simulink model "Vaja6_simulink"  (R2019b)
settings: Solver=FixedStepDiscrete  StartTime=0.0  StopTime=8  FixedStep=dT  RelTol=1e-3  EnableMultiTasking=on
values from neighbouring files (symbols this model uses):
  dT = 1/500    (= 0.002)    [initVR.m]    (also in trajectory.m = 0.00025)
  q0 = [0 0 0 0 90 0]'*pi/180    [initVR.m]    (also in trajectory.m)
undefined symbols (not defined in the file or in its folder): DiscIntNeverNeededParam, q2ZYXeul
libraries: simulink x2, xpcutilitieslib x2, dspnetwork x2, dspinverses x1
Description:
  | Real-Time Van der Pol Simulation
  | 
  | This demonstration shows a real-time version of the Simulink Van der Pol
  | simulation demo. This model does not need any external signals, so it does
  | not need any data acquisition hardware or driver. This makes the model ideal
  | for first experiments with Real-Time Windows Target, without need to
  | worry about proper I/O hardware configuration.
  | 
  | How to run this demo:
  | 
  |   1. Build the model using Tools -> Real-Time Workshop -> Build Model.
  |   2. Connect to the real-time code using Simulation -> Connect to target.
  |   3. Start the real-time execution using Simulation -> Start real-time code.
settings Model: EnablePacing=on  Creator=Houska  LastModifiedBy=student
settings DataIOCC: LimitDataPoints=on  SaveFormat=Array  SignalLoggingSaveFormat=ModelDataLogs  SaveOutput=off  SaveTime=off  ReturnWorkspaceOutputs=off  SignalLoggingName=logsOut
settings OptimizationCC: ExpressionDepthLimit=2147483647  InitFltsAndDblsToZero=on  LifeSpan=inf
settings DebuggingCC: SaveWithParameterizedLinksMsg=none  UnderspecifiedInitializationDetection=Classic  MergeDetectMultiDrivingBlocksExec=none  SignalResolutionControl=TryResolveAllWithWarning  MultiTaskDSMMsg=warning  MultiTaskCondExecSysMsg=none  FcnCallInpInsideContextMsg=warning  StateNameClashWarn=warning  SFUnexpectedBacktrackingDiag=warning  SFNoUnconditionalDefaultTransitionDiag=warning  SFExecutionAtInitializationDiag=none  ArithmeticOperatorsInVariantConditions=warning
settings HardwareCC: ProdBitPerPointer=32  ProdBitPerSizeT=32  ProdBitPerPtrDiffT=32  ProdLargestAtomicFloat=None  ProdWordSize=32  ProdHWDeviceType=32-bit Real-Time Windows Target
settings ModelReferenceCC: PropagateSignalLabelsOutOfModel=off
settings SFSimCC: SimUseLocalCustomCode=off  SimParseCustomCode=off  CustomCodeUndefinedFunction=UseInterfaceOnly
settings RTWCC: Description=Real-Time Windows Target  SystemTargetFile=rtwin.tlc  TemplateMakefile=rtwin.tmf  RTWUseLocalCustomCode=off
settings CodeAppCC: StateflowObjectComments=on
settings TargetCC: TargetFcnLib=ansi_tfl_tmw.mat  ModelReferenceCompliant=off  CompOptLevelCompliant=off  PreserveStateflowLocalDataDimensions=off
settings ConfigComp: CovMetricSettings=dw  CovHtmlReporting=on  CovSaveCumulativeToWorkspaceVar=on  CovSaveSingleToWorkspaceVar=on  CovExternalEMLEnable=off

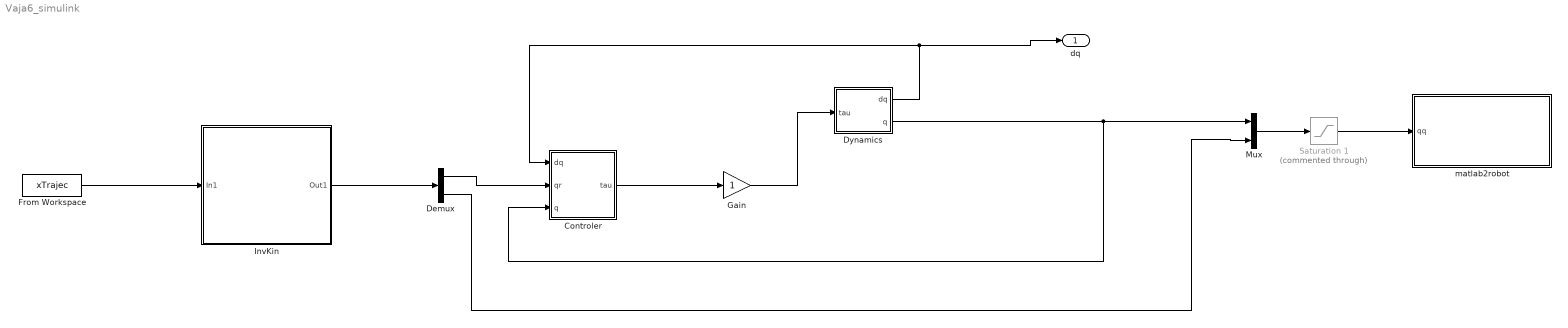
== system Vaja6_simulink ==
  Controler : Subsystem
  Demux : Demux  Outputs=2
  Dynamics : Subsystem
  From Workspace : FromWorkspace  VariableName=xTrajec  SampleTime=0
  Gain : Gain
  InvKin : Subsystem
  Mux : Mux  Inputs=2
  Saturation 1 : Saturate  Commented=through
  matlab2robot : Subsystem  mask{selUDP=Simulacija, slrt_ip='192.168.65.250', slrt_port=55555, sampleTime=dT}
      mask prompts: selUDP "Izvajanje programa:"; slrt_ip "Simulink Real Time IP:"; slrt_port "Simulink Real Time Port:"; sampleTime "Vzorcni cas:"
      mask init:
      | switch selUDP
      |     case 1
      |         enSim = 1;
      |         enRob = 0;
      |     case 2
      |         enSim = 0;
      |         enRob = 1;
      |     otherwise
      |         enSim = 0;
      |         enRob = 0;
      | end
      mask TypeOptions selUDP: Simulacija | Robot
  dq : Outport
  wires:
  Saturation 1/1 -> matlab2robot/1(qq)
  From Workspace/1 -> InvKin/1(In1)
  Dynamics/2(q) -> Mux/1, Controler/3(q)
  Controler/1(tau) -> Gain/1
  Dynamics/1(dq) -> Controler/1(dq), dq/1
  InvKin/1(Out1) -> Demux/1
  Demux/1 -> Controler/2(qr)
  Mux/1 -> Saturation 1/1
  Demux/2 -> Mux/2
  Gain/1 -> Dynamics/1(tau)

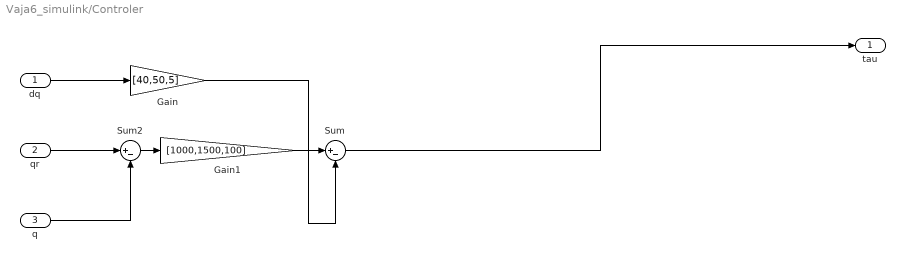
== system Vaja6_simulink/Controler ==
  dq : Inport
  qr : Inport  Port=2
  q : Inport  Port=3
  Gain : Gain  Gain=[40,50,5]
  Gain1 : Gain  Gain=[1000,1500,100]
  Sum : Sum  Inputs=|+-
  Sum2 : Sum  Inputs=|+-
  tau : Outport
  wires:
  Sum/1 -> tau/1
  Sum2/1 -> Gain1/1
  q/1 -> Sum2/2
  dq/1 -> Gain/1
  qr/1 -> Sum2/1
  Gain/1 -> Sum/2
  Gain1/1 -> Sum/1

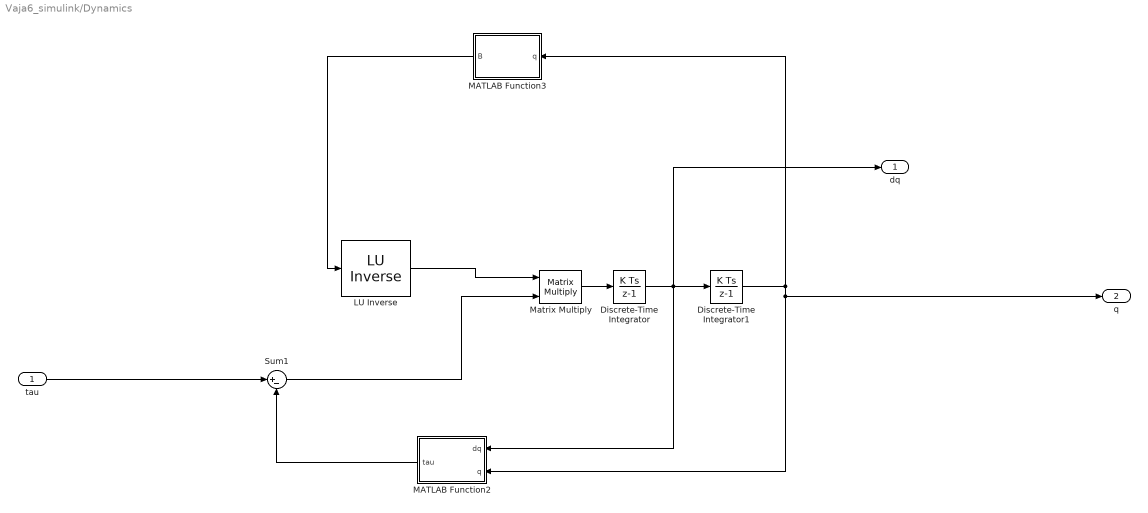
== system Vaja6_simulink/Dynamics ==
  tau : Inport
  " LU Inverse" : dspinverses/ LU Inverse
      settings: SourceProductName=DSP System Toolbox
  Discrete-Time Integrator : DiscreteIntegrator  InitialCondition=[0 0 0]  SampleTime=dT  ICPrevOutput=DiscIntNeverNeededParam  ICPrevScaledInput=DiscIntNeverNeededParam
  Discrete-Time Integrator1 : DiscreteIntegrator  InitialCondition=q0(1:3)  SampleTime=dT  ICPrevOutput=DiscIntNeverNeededParam  ICPrevScaledInput=DiscIntNeverNeededParam
  MATLAB Function2 : MATLAB Function  TreatAsAtomicUnit=on
  MATLAB Function3 : MATLAB Function  TreatAsAtomicUnit=on
  Matrix Multiply : Product  Multiplication=Matrix(*)
  Sum1 : Sum  Inputs=|+-
  dq : Outport
  q : Outport  Port=2
  wires:
  Discrete-Time Integrator/1 -> dq/1, Discrete-Time Integrator1/1, MATLAB Function2/1(dq)
  Discrete-Time Integrator1/1 -> q/1, MATLAB Function2/2(q), MATLAB Function3/1(q)
  Sum1/1 -> Matrix Multiply/2
  MATLAB Function3/1(B) -> " LU Inverse"/1
  " LU Inverse"/1 -> Matrix Multiply/1
  MATLAB Function2/1(tau) -> Sum1/2
  Matrix Multiply/1 -> Discrete-Time Integrator/1
  tau/1 -> Sum1/1

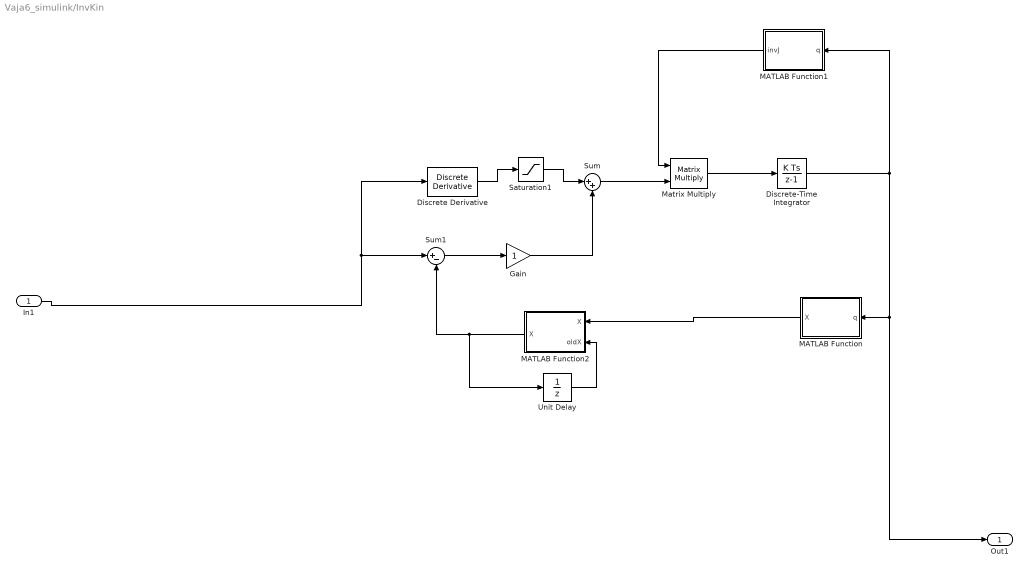
== system Vaja6_simulink/InvKin ==
  In1 : Inport
  Discrete Derivative : simulink/Discrete/Discrete Derivative  gainval=1.0  ICPrevScaledInput=0.0  OutMin=[]  OutMax=[]  OutDataType=fixdt(1, 16)  OutScaling=2^-10  DoSatur=off
  Discrete-Time Integrator : DiscreteIntegrator  InitialCondition=q0  SampleTime=dT  ICPrevOutput=DiscIntNeverNeededParam  ICPrevScaledInput=DiscIntNeverNeededParam
  Gain : Gain
  MATLAB Function : MATLAB Function  TreatAsAtomicUnit=on
  MATLAB Function1 : MATLAB Function  TreatAsAtomicUnit=on
  MATLAB Function2 : MATLAB Function  TreatAsAtomicUnit=on
  Matrix Multiply : Product  Multiplication=Matrix(*)
  Saturation1 : Saturate
  Sum : Sum  Inputs=|++
  Sum1 : Sum  Inputs=|+-
  Unit Delay : UnitDelay  InitialCondition=q2ZYXeul(q0)  SampleTime=-1  HasFrameUpgradeWarning=on
  Out1 : Outport
  wires:
  Sum1/1 -> Gain/1
  Saturation1/1 -> Sum/1
  MATLAB Function/1(X) -> MATLAB Function2/1("X ")
  Unit Delay/1 -> MATLAB Function2/2(oldX)
  MATLAB Function2/1(X) -> Unit Delay/1, Sum1/2
  Sum/1 -> Matrix Multiply/2
  Gain/1 -> Sum/2
  Matrix Multiply/1 -> Discrete-Time Integrator/1
  In1/1 -> Discrete Derivative/1, Sum1/1
  MATLAB Function1/1(invJ) -> Matrix Multiply/1
  Discrete-Time Integrator/1 -> Out1/1, MATLAB Function/1(q), MATLAB Function1/1(q)
  Discrete Derivative/1 -> Saturation1/1

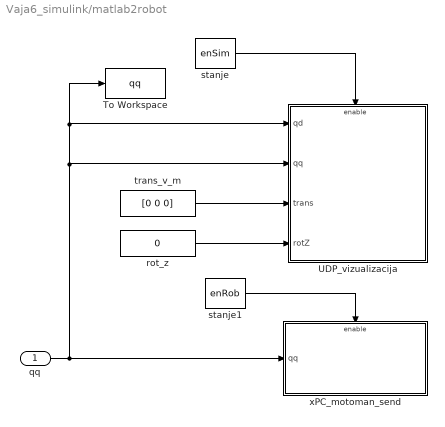
== system Vaja6_simulink/matlab2robot ==
  qq : Inport
  To Workspace : ToWorkspace  VariableName=qq  SampleTime=-1
  UDP_vizualizacija : Subsystem
  rot_z : Constant  Value=0
  stanje : Constant  Value=enSim  SampleTime=dT
  stanje1 : Constant  Value=enRob  SampleTime=dT
  trans_v_m : Constant  Value=[0 0 0]
  xPC_motoman_send : Subsystem  mask{IDSeje=rand(1), GetReady=1, slrt_ip1=slrt_ip, slrt_port1=slrt_port}
      mask prompts: IDSeje "IDSeje Function"; GetReady "GetReady Function"; slrt_ip1 "xPC Target IP"; slrt_port1 "xPC Target port"
      mask init:
      | %set_param([gcb,'/Send'],'remoteURL',slrt_ip1);
      | %set_param([gcb,'/Send'],'remotePort',num2str(slrt_port1));
      mask Callback slrt_port1: % set_param([gcb,'/Send'],'ipPort',slrt_port)
  wires:
  stanje/1 -> UDP_vizualizacija/Enable
  rot_z/1 -> UDP_vizualizacija/4(rotZ)
  trans_v_m/1 -> UDP_vizualizacija/3(trans)
  qq/1 -> To Workspace/1, UDP_vizualizacija/1(qd), UDP_vizualizacija/2(qq), xPC_motoman_send/1(qq)
  stanje1/1 -> xPC_motoman_send/Enable

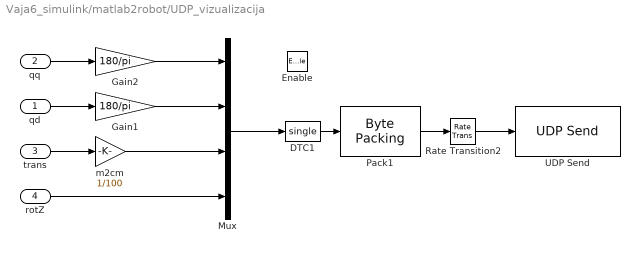
== system Vaja6_simulink/matlab2robot/UDP_vizualizacija ==
  qd : Inport
  qq : Inport  Port=2
  trans : Inport  Port=3
  rotZ : Inport  Port=4
  Enable : EnablePort  StatesWhenEnabling=reset
  DTC1 : DataTypeConversion  OutDataTypeStr=single
  Gain1 : Gain  Gain=180/pi
  Gain2 : Gain  Gain=180/pi
  Mux : Mux
  Pack1 : xpcutilitieslib/Byte Packing   MaskPackedDataType=uint8  MaskUnpackedDataTypes={'single'}  MaskAlignment=1
  Rate Transition2 : RateTransition
  UDP Send : dspnetwork/UDP Send  remoteURL='127.0.0.1'  remotePort=25300  localURL='0.0.0.0'  localPortSource=Automatically determine  localPort=-1  sampletime=-1  blockPlatform=[]  separateLengthPort=0
      settings: SourceProductName=Simulink
  m2cm : Gain  Gain=1/100
  wires:
  trans/1 -> m2cm/1
  Mux/1 -> DTC1/1
  m2cm/1 -> Mux/3
  rotZ/1 -> Mux/4
  qq/1 -> Gain2/1
  qd/1 -> Gain1/1
  Gain2/1 -> Mux/1
  Gain1/1 -> Mux/2
  Pack1/1 -> Rate Transition2/1
  Rate Transition2/1 -> UDP Send/1
  DTC1/1 -> Pack1/1

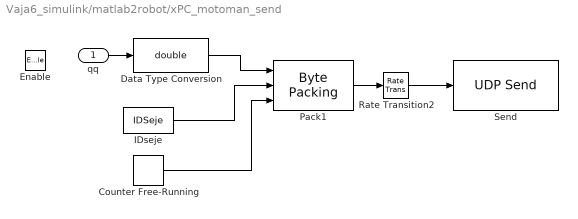
== system Vaja6_simulink/matlab2robot/xPC_motoman_send ==
  qq : Inport
  Enable : EnablePort  StatesWhenEnabling=reset
  Counter Free-Running : simulink/Sources/Counter Free-Running  NumBits=16  tsamp=-1
  Data Type Conversion : DataTypeConversion  OutDataTypeStr=double  SampleTime=dT
  IDseje : Constant  Value=IDSeje  SampleTime=dT
  Pack1 : xpcutilitieslib/Byte Packing   MaskPackedDataType=uint8  MaskUnpackedDataTypes={'double','double','uint16'}  MaskAlignment=1
  Rate Transition2 : RateTransition
  Send : dspnetwork/UDP Send  remoteURL='192.168.65.250'  remotePort=55555  localURL='0.0.0.0'  localPortSource=Automatically determine  localPort=-1  sampletime=-1  blockPlatform=[]  separateLengthPort=0
      settings: SourceProductName=Simulink
  wires:
  qq/1 -> Data Type Conversion/1
  IDseje/1 -> Pack1/2
  Data Type Conversion/1 -> Pack1/1
  Counter Free-Running/1 -> Pack1/3
  Pack1/1 -> Rate Transition2/1
  Rate Transition2/1 -> Send/1

== matlab function Vaja6_simulink/InvKin/MATLAB Function1 ==
  data: q input; invJ output
function invJ  = ijacZYXeul(q)

% q - Vrednost kotov v sklepih robota (vhod).
% invJ - Inverzna analiticna Jacobijeva matrika, kjer je orientacija
% predstavljena z ZYX Eulerjevimi koti (izhod).

% Izracun geometrijske Jacobijeve matrike (Jg).
Jg = jacobi0(q); %%% STUDENT %%%

% Izracun lege vrha robota z ZYX Eulerjevimi koti za opis orientacije.
X = q2ZYXeul(q); %%% STUDENT %%%

% Iz vektorja X izluscimo ustrezne komponente Eulerjevih kotov.
fi = X(4,1); %%% STUDENT %%%
theta = X(5,1); %%% STUDENT %%%
psi = X(6,1); %%% STUDENT %%%

% Izracun transformacijske matrike za pretvorbo iz geometrijske v
% analiticno Jacobijevo matriko.
Tr = [0, -sin(fi), cos(fi)*cos(theta); 
      0,  cos(fi), sin(fi)*cos(theta); 
      1,        0, -sin(theta)]; %%% STUDENT %%%
 
  
  Ja = [eye(3,3)  , zeros(3,3);
        zeros(3,3), Tr];
      
  
% Izracun inverzne analiticne Jacobijeve matrike.
invJ = inv(Jg)*Ja; %%% STUDENT %%%

end

== matlab function Vaja6_simulink/InvKin/MATLAB Function ==
  data: q input; X output
function X  = q2ZYXeul(q)

% q - Vektor kotnih spremenljivk robota (vhod).
% x - Lega vrha robota XYZ in orientacija z ZYX Eulerjevimi koti (izhod).

% Matrika lege vrha robota.
T6 = dirkinT6(dirkinA(q)); %%% STUDENT %%%

% Izluscimo ustrezne komponente rotacijske matrike.
r21 = T6(2, 1); %(vrstica, stolpec)
r31 = T6(3, 1); %%% STUDENT %%%
r32 = T6(3, 2); %%% STUDENT %%%
r33 = T6(3, 3); %%% STUDENT %%%
r11 = T6(1, 1); %%% STUDENT %%%

% Izracunamo ustrezne Eulerjeve kote.
fi = atan2(r21,r11); %%% STUDENT %%%
theta = atan2(-r31,sqrt(r32^2 + r33^2)); %%% STUDENT %%%
psi = atan2(r32,r33); %%% STUDENT %%%

% Orientacija vrha predstavljena z vektorjem treh ZYX Eulerjevih kotov.
ea = [fi; theta; psi];

% Lega vrha robota v smislu polozaja XYZ in orientacije predstavljene z
% ZYX Eulerjevimi koti.
X = [T6(1, 4); T6(2, 4); T6(3, 4); fi; theta; psi]; %%% STUDENT %%%

end

== matlab function Vaja6_simulink/Dynamics/MATLAB Function2 ==
  data: dq input; tau output; q input
function tau = tau3_q_dq(dq, q)

    % Funkcija izracuna navore v sklepih robota, ki so posledica delovanja 
    % Coriolisovih in gravitacijskih komponent ter posledica trenja.
    % Vhodni vektorji so polozaji v sklepih q in sklepne hitrosti dq.
    % Izhod funkcije je vektor sklepnih navorov tau.

    % Upostevamo pogoj za pospesek, ki deluje na bazo robota.
        ddp0 = [0 0 9.81]'; %Gravitacija                                           %%% STUDENT %%%

    % Upostevamo pogoj za kotne pospeske v sklepih.
        ddq = [0 0 0]';                                             %%% STUDENT %%%

    % Uporabimo funkcijo za izracun inverzne dinamike robota
    % za izracun navorov.
        tau = torque(ddq, dq, q, ddp0);                                             %%% STUDENT %%%
        
%tau3_q_dq([1,2,3]',[4,5,6]')

== matlab function Vaja6_simulink/Dynamics/MATLAB Function3 ==
  data: q input; B output
function B = inertia3(q)

    % Funkcija izracuna vztrajnostno matriko za robot s tremi segmenti.
    % Vhod je vektor kotov v sklepih q.

    % Inicializacijs vztrajnostne matrike.
        B = zeros(3,3);

    % Upostevamo pogoj za pospesek, ki deluje na bazo robota.
        ddp0 = [0 0 0]';                                            %%% STUDENT %%%

    % Upostevamo pogoj za kotne pospeske v sklepih.
        dq = [0 0 0]';                                              %%% STUDENT %%%

    
    % Izracunamo prvi stolpec vztrajnostne matrike B, pri cemer uporabimo
    % funkcijo za izracun inverzne dinamike robota za izracun navorov, 
    % ki predstavljajo stolpec matrike vztrajnosti.
        ddq = [1 0 0]';                                             %%% STUDENT %%%
        B(:,1) = torque(ddq, dq, q, ddp0);                                          %%% STUDENT %%%

    % Izracunamo drugi stolpec vztrajnostne matrike B.
        ddq = [0 1 0]';                                             %%% STUDENT %%%
        B(:,2) = torque(ddq, dq, q, ddp0);                                          %%% STUDENT %%%
        
    % Izracunamo tretji stolpec vztrajnostne matrike B.
        ddq = [0 0 1];                                             %%% STUDENT %%%
        B(:,3) = torque(ddq, dq, q, ddp0);                                          %%% STUDENT %%%
end

%inertia3([1, 2, 3]')

== matlab function Vaja6_simulink/InvKin/MATLAB Function2 ==
  data: X input; X output; oldX input
function X = skoki(X,oldX)

for i = 4:6
    if abs(X(i)-oldX(i)) >= pi
        X(i)=X(i)-sign(X(i)-oldX(i))*2*pi;
    end
end

        



%q = X1;
%if abs(q - oldX) >= pi
%    X = q - sign(q - oldX)*2*pi;

%else
%    X = q;

%end
